simulink model "A4_control_loop_nlin_c_model"  (Simulink 8.7)
settings: Solver=ode45  StartTime=0.0  StopTime=5  MaxStep=1e-3  RelTol=1e-3
values from neighbouring files (symbols this model uses):
  b_1 = 2.39e6    (= 2390000)    [a1_main.m]    (also in a2_main.m; a3_main.m; a4_main.m)
  c_oil = 36.5e6    (= 36500000)    [a1_main.m]    (also in a2_main.m; a3_main.m; a4_main.m)
  c_p = 75e6    (= 75000000)    [a1_main.m]    (also in a2_main.m; a3_main.m; a4_main.m)
  H = sum_H * lin_sys.b    [a2_main.m]    (also in a3_main.m; a4_main.m)
  K_I = 0.31    [a3_main.m]    (also in a4_main.m)
  K_M = 1/63000    (= 1.5873015873e-05)    [a1_main.m]    (also in a2_main.m; a3_main.m; a4_main.m)
  lin_sys = linmod('A1_Hydropulszylinder',zeros(3,1),0)    [a1_main.m]    (also in a2_main.m; a3_main.m; a4_main.m)
  m_g = m_k + m_p    (= 268.7)    [a1_main.m]    (also in a2_main.m; a3_main.m; a4_main.m)
  PHI = expm(Ta*lin_sys.a)    [a2_main.m]    (also in a3_main.m; a4_main.m)
  Ta = 15e-3    (= 0.015)    [a1_main.m]    (also in a2_main.m; a3_main.m; a4_main.m)
  u_max = 0.8    [a4_main.m]
undefined symbols (not defined in the file or in its folder): DiscIntNeverNeededParam
libraries: simulink x1
settings Model: Creator=jinyao  LastModifiedBy=jinyao
settings DataIOCC: LimitDataPoints=off  SaveFormat=Dataset
settings DebuggingCC: UnderspecifiedInitializationDetection=Simplified  MergeDetectMultiDrivingBlocksExec=error
settings HardwareCC: ProdBitPerPointer=64  ProdLargestAtomicFloat=Float  ProdIntDivRoundTo=Zero  ProdEndianess=LittleEndian  ProdWordSize=64  ProdHWDeviceType=Intel->x86-64 (Windows64)
settings ModelReferenceCC: PropagateSignalLabelsOutOfModel=on
settings ConfigComp: CovModelRefEnable=off

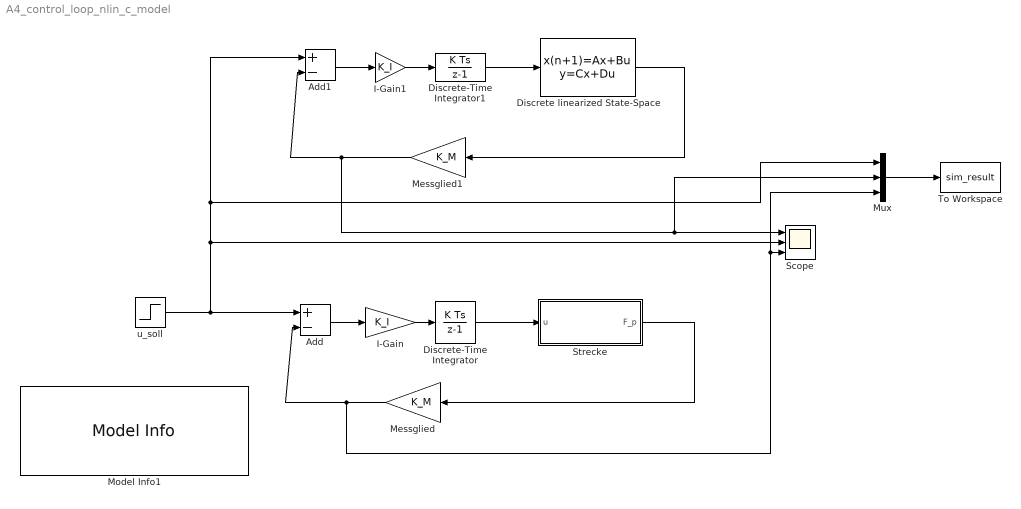
== system A4_control_loop_nlin_c_model ==
  Add : Sum  Inputs=+-
  Add1 : Sum  Inputs=+-
  Discrete linearized State-Space : DiscreteStateSpace  A=PHI  B=H  C=lin_sys.c  D=0  SampleTime=Ta
  Discrete-Time Integrator : DiscreteIntegrator  InitialConditionSetting=State (most efficient)  SampleTime=Ta  ICPrevOutput=DiscIntNeverNeededParam  ICPrevScaledInput=DiscIntNeverNeededParam
  Discrete-Time Integrator1 : DiscreteIntegrator  InitialConditionSetting=State (most efficient)  SampleTime=Ta  ICPrevOutput=DiscIntNeverNeededParam  ICPrevScaledInput=DiscIntNeverNeededParam
  I-Gain : Gain  Gain=K_I
  I-Gain1 : Gain  Gain=K_I
  Messglied : Gain  Gain=K_M
  Messglied1 : Gain  Gain=K_M
  Model Info1 : simulink/Model-Wide Utilities/Model Info  Frame=on  DisplayStringWithTags=|  HorizontalTextAlignment=Center  LeftAlignmentValue=0.5  SourceBlockDiagram=A4_control_loop_nlin_c_model  TagMaxNumber=20
      | %<ModelName>
      | 
      | MODSIM GRUPPE 11
      | 
      | Cao,Bozhi  Gao,Yue  Jia,Xuehua  Zhu,Jinyao
      | 
      | 14.06.2018
  Mux : Mux  Inputs=3
  Scope : Scope  NumInputPorts=3
  Strecke : Subsystem
  To Workspace : ToWorkspace  VariableName=sim_result  SaveFormat=Structure With Time  SampleTime=-1
  u_soll : Step  After=u_max  SampleTime=0
  wires:
  I-Gain/1 -> Discrete-Time Integrator/1
  Add/1 -> I-Gain/1
  Discrete-Time Integrator1/1 -> Discrete linearized State-Space/1
  Discrete linearized State-Space/1 -> Messglied1/1
  Messglied1/1 -> Mux/2, Scope/1, Add1/2
  Add1/1 -> I-Gain1/1
  I-Gain1/1 -> Discrete-Time Integrator1/1
  Strecke/1(F_p) -> Messglied/1
  u_soll/1 -> Mux/1, Add1/1, Scope/2, Add/1
  Messglied/1 -> Mux/3, Scope/3, Add/2
  Mux/1 -> To Workspace/1
  Discrete-Time Integrator/1 -> Strecke/1(u)

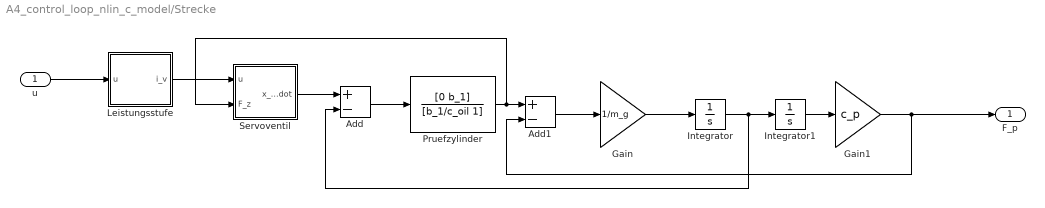
== system A4_control_loop_nlin_c_model/Strecke ==
  u : Inport
  Add : Sum  Inputs=+-
  Add1 : Sum  Inputs=+-
  Gain : Gain  Gain=1/m_g
  Gain1 : Gain  Gain=c_p
  Integrator : Integrator
  Integrator1 : Integrator
  Leistungsstufe : Subsystem
  Pruefzylinder : TransferFcn  Numerator=[0 b_1]  Denominator=[b_1/c_oil 1]
  Servoventil : Subsystem
  F_p : Outport
  wires:
  Leistungsstufe/1(i_v) -> Servoventil/1(u)
  Servoventil/1(x_oil_dot) -> Add/1
  Add/1 -> Pruefzylinder/1
  Add1/1 -> Gain/1
  Pruefzylinder/1 -> Servoventil/2(F_z), Add1/1
  Gain/1 -> Integrator/1
  Integrator1/1 -> Gain1/1
  Integrator/1 -> Add/2, Integrator1/1
  Gain1/1 -> F_p/1, Add1/2
  u/1 -> Leistungsstufe/1(u)

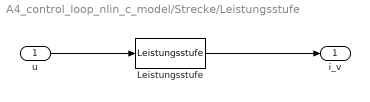
== system A4_control_loop_nlin_c_model/Strecke/Leistungsstufe ==
  u : Inport
  Leistungsstufe : MATLABFcn  MATLABFcn=Leistungsstufe  OutputDimensions=1  OutputSignalType=real
  i_v : Outport
  wires:
  Leistungsstufe/1 -> i_v/1
  u/1 -> Leistungsstufe/1

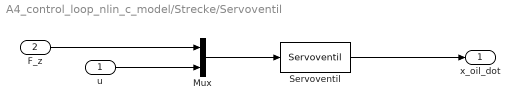
== system A4_control_loop_nlin_c_model/Strecke/Servoventil ==
  u : Inport
  F_z : Inport  Port=2
  Mux : Mux  Inputs=2
  Servoventil : MATLABFcn  MATLABFcn=Servoventil  OutputDimensions=1  OutputSignalType=real
  x_oil_dot : Outport
  wires:
  Servoventil/1 -> x_oil_dot/1
  u/1 -> Mux/2
  Mux/1 -> Servoventil/1
  F_z/1 -> Mux/1
